simulink model "sensor_block_together"  (Simulink 7.4)
settings: Solver=FixedStepDiscrete  StartTime=0  StopTime=inf  FixedStep=0.01  RelTol=1e-3
settings Model: Creator=kthwsnt  LastModifiedBy=aitorhh
settings SolverCC: PositivePriorityOrder=on
settings DataIOCC: LimitDataPoints=off  SaveOutput=off  SignalLogging=off  SaveTime=off
settings OptimizationCC: InitFltsAndDblsToZero=on
settings SimEventsCC: propDiagAttribOutput=1  propDiagFcnCallOutput=1  propDiagStatOutput=0

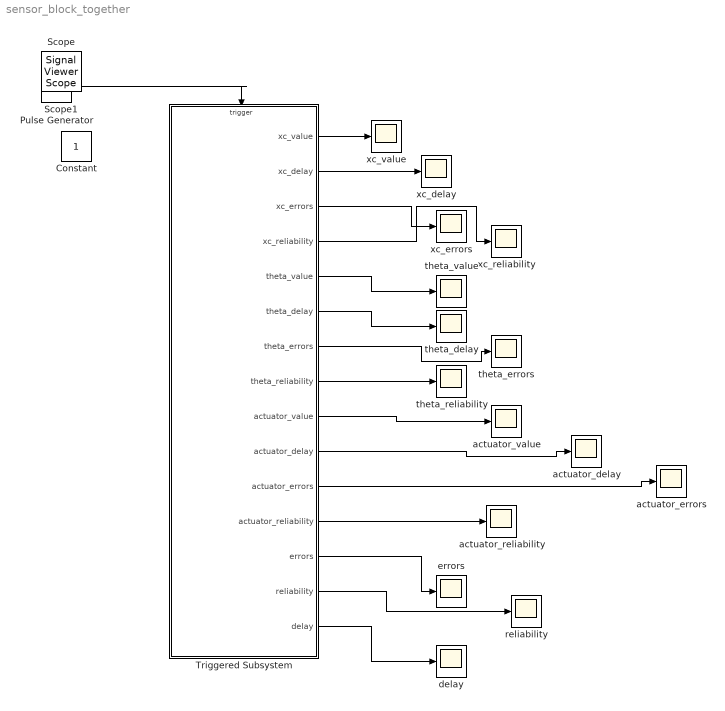
== system sensor_block_together ==
  Pulse Generator : DiscretePulseGenerator  Amplitude=1  Period=1  PulseWidth=1  PhaseDelay=0  SampleTime=1
  Triggered Subsystem : Subsystem  TreatAsAtomicUnit=on
  actuator_delay : Scope
      settings: TimeRange=1000  YMin=-1  YMax=1  SaveName=ScopeData16
  actuator_errors : Scope
      settings: TimeRange=1000  YMin=-1  YMax=1  SaveName=ScopeData22
  actuator_reliability : Scope
      settings: TimeRange=1000  YMin=-1  YMax=1  SaveName=ScopeData23
  actuator_value : Scope
      settings: TimeRange=1000  YMin=-1  YMax=1  SaveName=ScopeData17
  delay : Scope
      settings: TimeRange=1000  YMin=360  YMax=520  SaveName=ScopeData2
  errors : Scope
      settings: TimeRange=100  YMin=-1  YMax=1
  reliability : Scope
      settings: TimeRange=1000  YMin=0.95  YMax=1.05
  theta_delay : Scope
      settings: TimeRange=1000  YMin=0  YMax=100  SaveName=ScopeData18
  theta_errors : Scope
      settings: TimeRange=1000  YMin=-1  YMax=1  SaveName=ScopeData24
  theta_reliability : Scope
      settings: TimeRange=1000  YMin=-1  YMax=1  SaveName=ScopeData25
  theta_value : Scope
      settings: TimeRange=1000  YMin=0  YMax=450  SaveName=ScopeData19
  xc_delay : Scope
      settings: TimeRange=1000  YMin=3  YMax=21  SaveName=ScopeData20
  xc_errors : Scope
      settings: TimeRange=1000  YMin=-1  YMax=1  SaveName=ScopeData26
  xc_reliability : Scope
      settings: TimeRange=1000  YMin=0  YMax=1  SaveName=ScopeData27  MaxDataPoints=500000
  xc_value : Scope
      settings: TimeRange=1000  YMin=-1  YMax=1  SaveName=ScopeData21
  Constant : Constant  IOType=siggen  OutDataType=sfix(16)  OutScaling=2^0
  Scope : SignalViewerScope  IOType=viewer  RefreshTime=0.035000
      settings: YMin=4427  YMax=4893
  Scope1 : SignalViewerScope  IOType=viewer  RefreshTime=0.035000
      settings: YMin=0  YMax=1
  wires:
  Pulse Generator/1 -> Triggered Subsystem/Trigger
  Triggered Subsystem/1(xc_value) -> xc_value/1
  Triggered Subsystem/2(xc_delay) -> xc_delay/1
  Triggered Subsystem/3(xc_errors) -> xc_errors/1
  Triggered Subsystem/4(xc_reliability) -> xc_reliability/1
  Triggered Subsystem/5(theta_value) -> theta_value/1
  Triggered Subsystem/6(theta_delay) -> theta_delay/1
  Triggered Subsystem/7(theta_errors) -> theta_errors/1
  Triggered Subsystem/8(theta_reliability) -> theta_reliability/1
  Triggered Subsystem/9(actuator_value) -> actuator_value/1
  Triggered Subsystem/10(actuator_delay) -> actuator_delay/1
  Triggered Subsystem/11(actuator_errors) -> actuator_errors/1
  Triggered Subsystem/12(actuator_reliability) -> actuator_reliability/1
  Triggered Subsystem/14(reliability) -> reliability/1
  Triggered Subsystem/13(errors) -> errors/1
  Triggered Subsystem/15(delay) -> delay/1

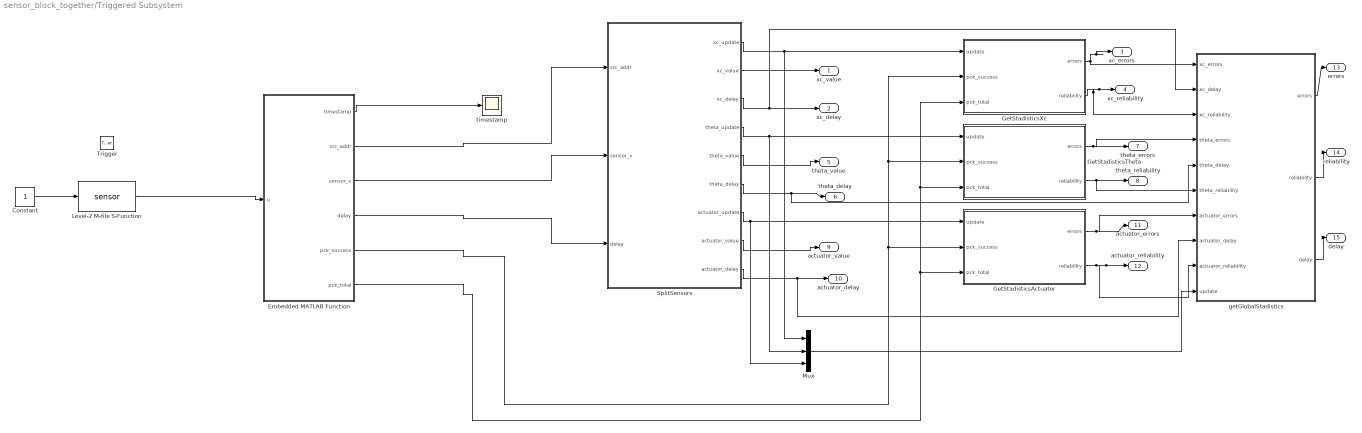
== system sensor_block_together/Triggered Subsystem ==
  Trigger : TriggerPort
  Constant : Constant  OutDataType=fixdt(1, 16)  OutScaling=2^0
  Embedded MATLAB Function : Stateflow chart
  GetStadisticsActuator : Stateflow chart
  GetStadisticsTheta : Stateflow chart
  GetStadisticsXc : Stateflow chart
  Level-2 M-file S-Function : M-S-Function  FunctionName=sensor
  Mux : Mux  Inputs=3
  SplitSensors : Stateflow chart
  getGlobalStadistics : Stateflow chart
  timestamp : Scope
      settings: TimeRange=1000  YMin=-1  YMax=1  SaveName=ScopeData3
  xc_value : Outport  OutDataType=fixdt(1, 16)  OutScaling=2^0
  xc_delay : Outport  Port=2  OutDataType=fixdt(1, 16)  OutScaling=2^0
  xc_errors : Outport  Port=3  OutDataType=fixdt(1, 16)  OutScaling=2^0
  xc_reliability : Outport  Port=4  OutDataType=fixdt(1, 16)  OutScaling=2^0
  theta_value : Outport  Port=5  OutDataType=fixdt(1, 16)  OutScaling=2^0
  theta_delay : Outport  Port=6  OutDataType=fixdt(1, 16)  OutScaling=2^0
  theta_errors : Outport  Port=7  OutDataType=fixdt(1, 16)  OutScaling=2^0
  theta_reliability : Outport  Port=8  OutDataType=fixdt(1, 16)  OutScaling=2^0
  actuator_value : Outport  Port=9  OutDataType=fixdt(1, 16)  OutScaling=2^0
  actuator_delay : Outport  Port=10  OutDataType=fixdt(1, 16)  OutScaling=2^0
  actuator_errors : Outport  Port=11  OutDataType=fixdt(1, 16)  OutScaling=2^0
  actuator_reliability : Outport  Port=12  OutDataType=fixdt(1, 16)  OutScaling=2^0
  errors : Outport  Port=13  OutDataType=fixdt(1, 16)  OutScaling=2^0
  reliability : Outport  Port=14  OutDataType=fixdt(1, 16)  OutScaling=2^0
  delay : Outport  Port=15  OutDataType=fixdt(1, 16)  OutScaling=2^0
  wires:
  Constant/1 -> Level-2 M-file S-Function/1
  Level-2 M-file S-Function/1 -> Embedded MATLAB Function/1(u)
  Embedded MATLAB Function/2(src_addr) -> SplitSensors/1(src_addr)
  SplitSensors/3(xc_delay) -> getGlobalStadistics/2(xc_delay), xc_delay/1
  SplitSensors/5(theta_value) -> theta_value/1
  SplitSensors/6(theta_delay) -> getGlobalStadistics/5(theta_delay), theta_delay/1
  SplitSensors/8(actuator_value) -> actuator_value/1
  SplitSensors/9(actuator_delay) -> getGlobalStadistics/8(actuator_delay), actuator_delay/1
  Embedded MATLAB Function/4(delay) -> SplitSensors/3(delay)
  Embedded MATLAB Function/3(sensor_v) -> SplitSensors/2(sensor_v)
  SplitSensors/1(xc_update) -> GetStadisticsXc/1(update), Mux/1
  GetStadisticsXc/2(reliability) -> getGlobalStadistics/3(xc_reliability), xc_reliability/1
  Embedded MATLAB Function/6(pck_total) -> GetStadisticsXc/3(pck_total), GetStadisticsTheta/3(pck_total), GetStadisticsActuator/3(pck_total)
  Embedded MATLAB Function/5(pck_success) -> GetStadisticsXc/2(pck_success), GetStadisticsTheta/2(pck_success), GetStadisticsActuator/2(pck_success)
  SplitSensors/4(theta_update) -> GetStadisticsTheta/1(update), Mux/2
  SplitSensors/7(actuator_update) -> GetStadisticsActuator/1(update), Mux/3
  GetStadisticsTheta/2(reliability) -> getGlobalStadistics/6(theta_reliability), theta_reliability/1
  GetStadisticsTheta/1(errors) -> getGlobalStadistics/4(theta_errors), theta_errors/1
  GetStadisticsActuator/1(errors) -> getGlobalStadistics/7(actuator_errors), actuator_errors/1
  GetStadisticsActuator/2(reliability) -> getGlobalStadistics/9(actuator_reliability), actuator_reliability/1
  Mux/1 -> getGlobalStadistics/10(update)
  GetStadisticsXc/1(errors) -> getGlobalStadistics/1(xc_errors), xc_errors/1
  getGlobalStadistics/1(errors) -> errors/1
  Embedded MATLAB Function/1(timestamp) -> timestamp/1
  SplitSensors/2(xc_value) -> xc_value/1
  getGlobalStadistics/2(reliability) -> reliability/1
  getGlobalStadistics/3(delay) -> delay/1

== matlab function Triggered Subsystem/GetStadisticsTheta ==
  data: update input double; pck_success input double; pck_total input double; errors output double; reliability output double
function [errors, reliability ] = ...
    getStadistics (update, pck_success,  pck_total)
%#eml
% 
persistent errors_window ...    %vector that contains the number of errors
    item ...                    %index of the vector
    pckTotalTrack ...           % vector that contains the number of total packets
    prevTotalPackets ...        % previous number of total packets to check if we have received a new one
    prevErrors;                 % previous number of errors

SLIDING_WINDOW = 50;

% First initialization of the variables
if isempty(item)
    errors_window = zeros(SLIDING_WINDOW, 1);
    pckTotalTrack = zeros(SLIDING_WINDOW, 1);
    item = 1;
    prevErrors = pck_total - pck_success;
    prevTotalPackets = pck_total;
end


    newPacket =  prevTotalPackets ~= pck_total;

if (update && newPacket)
    currentItem = mod(item + 1, SLIDING_WINDOW+1);
    if currentItem == 0
        currentItem = 1;
    end
    
    % It could be that the number of received packets
    % is not the total packets sent, so we need
    % to keep track of it.
    pckTotalTrack(currentItem) = pck_total - prevTotalPackets;
    if pckTotalTrack(currentItem) <= 0
        pckTotalTrack(currentItem) = 1;
    end %when we restart the counters
    
    
    % if the previous errors in less than the actual value
    % it means that we get a need error
    errors_window(currentItem) = (pck_total - pck_success) - prevErrors;
    %%in case....
    if errors_window(currentItem) < 0
        errors_window(currentItem) = 0;
    end %when we restart the counters
    
    
    % update with the current data
    prevErrors = pck_total - pck_success;
    prevTotalPackets = pck_total;
    item = currentItem;
end

%
% Map the outputs
errors = errors_window(item);
if sum(pckTotalTrack) == 0 
    reliability = 0;
else
    reliability = 1-sum(errors_window)/(sum(pckTotalTrack));
end

== matlab function Triggered Subsystem/Embedded MATLAB Function ==
  data: u input double; timestamp output double; src_addr output double; sensor_v output double; delay output double; pck_success output double; pck_total output double
function [timestamp, src_addr, sensor_v, delay, pck_success, pck_total ] = parsePacket(u)

% 02    0f     61 88   e7     34 12     03 00      00 00    00 13    04 e3    0f ff    69    c9     00        c0  2d  40  58 
% 02    0f     61 88   d2     34 12     03 00      00 00    00 00    00 00    07 ff    69    c2     84        32 8d de 02 
% 02    0f     61 88   be     34 12     03 00      00 00    00 00    00 00    07 ff    67    ca     00        c4 f0 8d 03 

% id| length|        |seqnum|  PANID  | Src adr | Dst addr | xc    | theta  |  u_out  | lqi | rssi| mhrLen | timestamp
%           
%#eml
% 02   0f     61 88    9f     34 12     00 00      02 00     00 00    00 4b      00 4b   02 04    6b    c2     00      ba 15 28 00 
% 02   11     61 88    7b     34 12     00 00      02 00     ff ff    00 23      00 00   05 84    6c    e0     11      a0 b8 dc 3d 

% id| length|        |seqnum|  PANID  | Dest adr | Src addr | xc    | total |  success  | delay | lqi | rssi| mhrLen | timestamp

l=length(u);
%
% packet information
%

seq_num = u(5);
pan_id = bitor(bitshift(uint16(u(7)),8), uint16(u(6)));
dst_addr = bitor(bitshift(uint16(u(9)),8), uint16(u(8)));
src_addr= bitor(bitshift(uint16(u(11)),8), uint16(u(10)));

%
% Sensors and control voltage
%
% xc_sensor=bitor(bitshift(uint16(u(14)),8), uint16(u(15)))*9.2E-5;
% theta_sensor=bitor(bitshift(uint16(u(12)),8), uint16(u(13))) / 1024.0 * 2 * 3.14159265;
% u_control = bitor(bitshift(uint16(u(16)),8), uint16(u(17)));
% u_control = (u_control / 1638) * 4.8 -6;

% Sensor values
sensor_v = bitor(bitshift(uint16(u(12)),8), uint16(u(13)));
pck_total = bitor(bitshift(uint16(u(14)),8), uint16(u(15)));
pck_success = bitor(bitshift(uint16(u(16)),8), uint16(u(17)));

%pck_total = uint8(u(14));
%pck_success = uint8(u(15));
delay = bitor(bitshift(uint16(u(18)),8), uint16(u(19)));

%
% Timestamps and more packet information
%
lqi=uint16(u(l-6));
rssi=uint16(u(l-5));

timestamp1 = bitor(bitshift(uint32(u(l-1)),24), bitshift(uint32(u(l-2)),16) );
timestamp2 = bitor(bitshift(uint32(u(l-3)),8), uint32(u(l-4) ));
timestamp = bitor(timestamp1, timestamp2)*16E-3; %%in ms

== matlab function Triggered Subsystem/SplitSensors ==
  data: xc_update output double; src_addr input double; xc_value output double; xc_delay output double; sensor_v input double; delay input double; theta_update output double; theta_value output double; theta_delay output double; actuator_update output double; actuator_value output double; actuator_delay output double
function [xc_update, xc_value, xc_delay, theta_update, theta_value, theta_delay, ...
        actuator_update, actuator_value, actuator_delay] = ...
        splitSensors(src_addr, sensor_v, delay)
%#eml
% 
persistent xc_value_p xc_delay_p ...
     theta_value_p theta_delay_p ...
     actuator_value_p actuator_delay_p;  
COORDINATOR_ADDRESS = 0;
XCART_ADDRESS = 1;
TPENDULUM_ADDRESS = 2;

TIME_SYMBOL = 1/(2*32678)*1E3;

NUMBER_LINKS = 2;
NUMBER_SENSORS = 2;


% First initialization of the variables
if isempty(xc_value_p)
    
    xc_value_p = double(0);
    xc_delay_p = double(0);
    
    theta_value_p = double(0);
    theta_delay_p = double(0);
    
    actuator_value_p = double(0);
    actuator_delay_p = double(0);

end
xc_update = false;
theta_update = false;
actuator_update = false;
    if ( src_addr <= (NUMBER_SENSORS + NUMBER_LINKS - 1) &&  src_addr > 0 )
        %
        % SENSOR ---- > COORDINATOR
        %
        
        % Set the new values for the desired sensors
        if src_addr == XCART_ADDRESS
            
            xc_value_p = double(sensor_v);
            xc_delay_p = double(delay);
            xc_update = true;
            
        elseif src_addr == TPENDULUM_ADDRESS
           
            theta_value_p = double(sensor_v);
            theta_delay_p = double(delay);
            theta_update = true;
            
        elseif src_addr == COORDINATOR_ADDRESS
            %
            % COORDIANTOR ---- > ACTUATOR
            %
            actuator_value_p = double(sensor_v);
            actuator_delay_p = double(delay);
            actuator_update = true;
        end
    end

xc_value = xc_value_p * 9.2E-5;
xc_delay = xc_delay_p * TIME_SYMBOL;

theta_value = (theta_value_p / 1024.0) * 2 * 3.14159265;
theta_delay = theta_delay_p  * TIME_SYMBOL;

actuator_value = actuator_value_p;
actuator_delay = actuator_delay_p * TIME_SYMBOL;

== matlab function Triggered Subsystem/GetStadisticsXc ==
  data: update input double; pck_success input double; pck_total input double; errors output double; reliability output double
function [errors, reliability ] = ...
    getStadistics (update, pck_success,  pck_total)
%#eml
% 
persistent errors_window ...    %vector that contains the number of errors
    item ...                    %index of the vector
    pckTotalTrack ...           % vector that contains the number of total packets
    prevTotalPackets ...        % previous number of total packets to check if we have received a new one
    prevErrors;                 % previous number of errors

SLIDING_WINDOW = 50;

% First initialization of the variables
if isempty(item)
    errors_window = zeros(SLIDING_WINDOW, 1);
    pckTotalTrack = zeros(SLIDING_WINDOW, 1);
    item = 1;
    prevErrors = pck_total - pck_success;
    prevTotalPackets = pck_total;
end


    newPacket =  prevTotalPackets ~= pck_total;

if (update && newPacket)
    currentItem = mod(item + 1, SLIDING_WINDOW+1);
    if currentItem == 0
        currentItem = 1;
    end
    
    % It could be that the number of received packets
    % is not the total packets sent, so we need
    % to keep track of it.
    pckTotalTrack(currentItem) = pck_total - prevTotalPackets;
    if pckTotalTrack(currentItem) <= 0
        pckTotalTrack(currentItem) = 1;
    end %when we restart the counters
    
    
    % if the previous errors in less than the actual value
    % it means that we get a need error
    errors_window(currentItem) = (pck_total - pck_success) - prevErrors;
    %%in case....
    if errors_window(currentItem) < 0
        errors_window(currentItem) = 0;
    end %when we restart the counters
    
    
    % update with the current data
    prevErrors = pck_total - pck_success;
    prevTotalPackets = pck_total;
    item = currentItem;
end

%
% Map the outputs
errors = errors_window(item);
if sum(pckTotalTrack) == 0 
    reliability = 0;
else
    reliability = 1-sum(errors_window)/(sum(pckTotalTrack));
end

== matlab function Triggered Subsystem/GetStadisticsActuator ==
  data: update input double; pck_success input double; pck_total input double; errors output double; reliability output double
function [errors, reliability ] = ...
    getStadistics (update, pck_success,  pck_total)
%#eml
% 
persistent errors_window ...    %vector that contains the number of errors
    item ...                    %index of the vector
    pckTotalTrack ...           % vector that contains the number of total packets
    prevTotalPackets ...        % previous number of total packets to check if we have received a new one
    prevErrors;                 % previous number of errors

SLIDING_WINDOW = 50;

% First initialization of the variables
if isempty(item)
    errors_window = zeros(SLIDING_WINDOW, 1);
    pckTotalTrack = zeros(SLIDING_WINDOW, 1);
    item = 1;
    prevErrors = pck_total - pck_success;
    prevTotalPackets = pck_total;
end


    newPacket =  prevTotalPackets ~= pck_total;

if (update && newPacket)
    currentItem = mod(item + 1, SLIDING_WINDOW+1);
    if currentItem == 0
        currentItem = 1;
    end
    
    % It could be that the number of received packets
    % is not the total packets sent, so we need
    % to keep track of it.
    pckTotalTrack(currentItem) = pck_total - prevTotalPackets;
    if pckTotalTrack(currentItem) <= 0
        pckTotalTrack(currentItem) = 1;
    end %when we restart the counters
    
    
    % if the previous errors in less than the actual value
    % it means that we get a need error
    errors_window(currentItem) = (pck_total - pck_success) - prevErrors;
    %%in case....
    if errors_window(currentItem) < 0
        errors_window(currentItem) = 0;
    end %when we restart the counters
    
    
    % update with the current data
    prevErrors = pck_total - pck_success;
    prevTotalPackets = pck_total;
    item = currentItem;
end

%
% Map the outputs
errors = errors_window(item);
if sum(pckTotalTrack) == 0 
    reliability = 0;
else
    reliability = 1-sum(errors_window)/(sum(pckTotalTrack));
end

== matlab function Triggered Subsystem/getGlobalStadistics ==
  data: xc_errors input double; xc_delay input double; xc_reliability input double; errors output double; reliability output double; theta_errors input double; theta_delay input double; theta_reliability input double; actuator_errors input double; actuator_delay input double; actuator_reliability input double; delay output double; update input double
function [errors, reliability, delay] = ...
    getStadistics (xc_errors, xc_delay, xc_reliability, ...
    theta_errors, theta_delay, theta_reliability, ...
    actuator_errors, actuator_delay, actuator_reliability, update)
%#eml
% 

LEARNING_WINDOW = 50;

persistent checkLinks idx;

%% detect how many links do we 
if isempty(checkLinks)
    samples =0;
    checkLinks = zeros(length(update), 1); 
    idx = 1;
end
if idx < LEARNING_WINDOW
  for i=1:length(checkLinks)
      if update(i) == 1
          checkLinks(i) = 1;
      end
  end
  idx = idx +1;
end

errors = xc_errors + theta_errors + actuator_errors;
reliability = (xc_reliability + theta_reliability + actuator_reliability)/sum(checkLinks);
delay = (xc_delay + theta_delay + actuator_delay)/sum(checkLinks);
